simulink model "Fly_By_Wire_Logical_Architecture"  (R2025a)
settings: Solver=VariableStepAuto  StartTime=0.0  StopTime=10.0  RelTol=1e-3
(part 1 of 2)
settings Model: Creator=annic  LastModifiedBy=annic

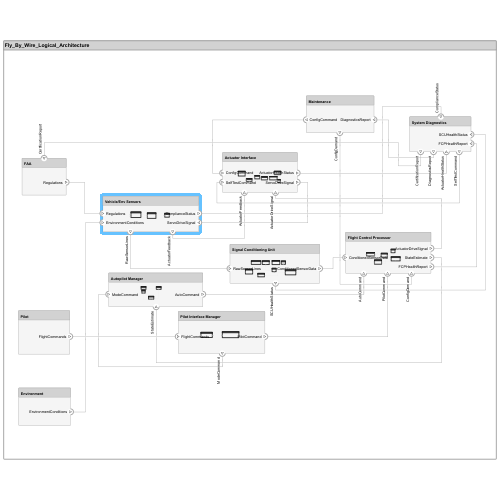
[thumbnail: Simulink's stored preview of the top-level diagram]
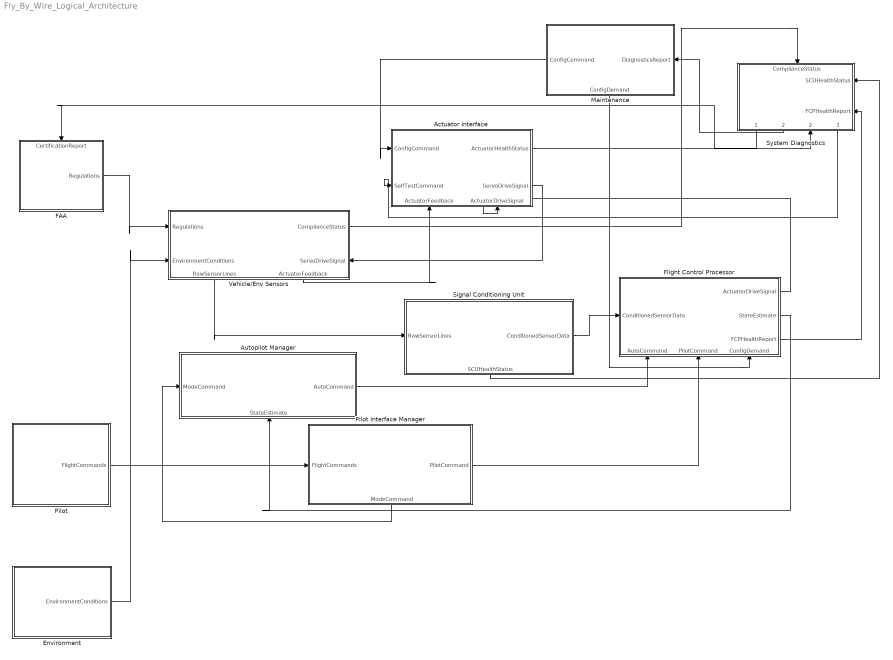
== system Fly_By_Wire_Logical_Architecture ==
  Actuator Interface : Subsystem
      settings: PortSchema="{\"entries\":[{\"content\":{\"headerSize\":26,\"margin\":15,\"minimumSpacing\":25,\"sides\":[{\"content\":{\"connectorIds\":[\"In3\",\"In1\"]},\"type\":\"ConnectorPlacement.EquallySpacedRectSide\",\"uuid\":\"65641699-9f7d-4c29-a70e-9e8ac59d97d8\"},{\"content\":{\"connectorIds\":[\"Out1\",\"Out2\"],\"side\":\"RIGHT\"},\"type\":\"ConnectorPlacement.EquallySpacedRectSide\",\"uuid\":\"1bd5edf9-dcd5-4263-91ef-6bf36c773327\"},{\"content\":{\"side\":\"TOP\"},\"type\":\"ConnectorPlacement.EquallySpacedRectSide\",\"uuid\":\"e3031d72-1a7c-40a3-b76e-c1b9cc4f41a2\"},{\"content\":{\"connectorIds\":[\"In2\",\"In4\"],\"side\":\"BOTTOM\"},\"type\":\"ConnectorPlacement.EquallySpacedRectSide\",\"uuid\":\"36dfb4ef-dbe8-4037-a31c-a1fb1d1c9c8b\"}]},\"type\":\"ConnectorPlacement.EquallySpacedConnector\",\"uuid\":\"735ff59d-d504-4a4c-a5dd-88c988b53692\"}],\"packageUris\":[\"http://schema.mathworks.com/mf0/Connector/R2020b\"],\"version\":\"1.0\"}"
  Autopilot Manager : Subsystem
      settings: PortSchema="{\"entries\":[{\"content\":{\"headerSize\":26,\"margin\":15,\"minimumSpacing\":25,\"sides\":[{\"content\":{\"connectorIds\":[\"In2\"]},\"type\":\"ConnectorPlacement.EquallySpacedRectSide\",\"uuid\":\"65641699-9f7d-4c29-a70e-9e8ac59d97d8\"},{\"content\":{\"connectorIds\":[\"Out1\"],\"side\":\"RIGHT\"},\"type\":\"ConnectorPlacement.EquallySpacedRectSide\",\"uuid\":\"1bd5edf9-dcd5-4263-91ef-6bf36c773327\"},{\"content\":{\"side\":\"TOP\"},\"type\":\"ConnectorPlacement.EquallySpacedRectSide\",\"uuid\":\"e3031d72-1a7c-40a3-b76e-c1b9cc4f41a2\"},{\"content\":{\"connectorIds\":[\"In1\"],\"side\":\"BOTTOM\"},\"type\":\"ConnectorPlacement.EquallySpacedRectSide\",\"uuid\":\"52da988e-5309-44fa-8186-16f50d2bf4d2\"}]},\"type\":\"ConnectorPlacement.EquallySpacedConnector\",\"uuid\":\"735ff59d-d504-4a4c-a5dd-88c988b53692\"}],\"packageUris\":[\"http://schema.mathworks.com/mf0/Connector/R2020b\"],\"version\":\"1.0\"}"
  Environment : Subsystem
      settings: PortSchema="{\"entries\":[{\"content\":{\"headerSize\":26,\"margin\":15,\"minimumSpacing\":25,\"sides\":[{\"content\":{},\"type\":\"ConnectorPlacement.EquallySpacedRectSide\",\"uuid\":\"65641699-9f7d-4c29-a70e-9e8ac59d97d8\"},{\"content\":{\"connectorIds\":[\"Out1\"],\"side\":\"RIGHT\"},\"type\":\"ConnectorPlacement.EquallySpacedRectSide\",\"uuid\":\"1bd5edf9-dcd5-4263-91ef-6bf36c773327\"},{\"content\":{\"side\":\"TOP\"},\"type\":\"ConnectorPlacement.EquallySpacedRectSide\",\"uuid\":\"e3031d72-1a7c-40a3-b76e-c1b9cc4f41a2\"}]},\"type\":\"ConnectorPlacement.EquallySpacedConnector\",\"uuid\":\"735ff59d-d504-4a4c-a5dd-88c988b53692\"}],\"packageUris\":[\"http://schema.mathworks.com/mf0/Connector/R2020b\"],\"version\":\"1.0\"}"
  FAA : Subsystem
      settings: PortSchema="{\"entries\":[{\"content\":{\"headerSize\":26,\"margin\":15,\"minimumSpacing\":25,\"sides\":[{\"content\":{},\"type\":\"ConnectorPlacement.EquallySpacedRectSide\",\"uuid\":\"65641699-9f7d-4c29-a70e-9e8ac59d97d8\"},{\"content\":{\"connectorIds\":[\"Out1\"],\"side\":\"RIGHT\"},\"type\":\"ConnectorPlacement.EquallySpacedRectSide\",\"uuid\":\"1bd5edf9-dcd5-4263-91ef-6bf36c773327\"},{\"content\":{\"connectorIds\":[\"In1\"],\"side\":\"TOP\"},\"type\":\"ConnectorPlacement.EquallySpacedRectSide\",\"uuid\":\"e3031d72-1a7c-40a3-b76e-c1b9cc4f41a2\"}]},\"type\":\"ConnectorPlacement.EquallySpacedConnector\",\"uuid\":\"735ff59d-d504-4a4c-a5dd-88c988b53692\"}],\"packageUris\":[\"http://schema.mathworks.com/mf0/Connector/R2020b\"],\"version\":\"1.0\"}"
  Flight Control Processor : Subsystem
      settings: PortSchema="{\"entries\":[{\"content\":{\"headerSize\":26,\"margin\":15,\"minimumSpacing\":25,\"sides\":[{\"content\":{\"connectorIds\":[\"In4\"]},\"type\":\"ConnectorPlacement.EquallySpacedRectSide\",\"uuid\":\"65641699-9f7d-4c29-a70e-9e8ac59d97d8\"},{\"content\":{\"connectorIds\":[\"Out1\",\"Out2\",\"Out3\"],\"side\":\"RIGHT\"},\"type\":\"ConnectorPlacement.EquallySpacedRectSide\",\"uuid\":\"1bd5edf9-dcd5-4263-91ef-6bf36c773327\"},{\"content\":{\"side\":\"TOP\"},\"type\":\"ConnectorPlacement.EquallySpacedRectSide\",\"uuid\":\"e3031d72-1a7c-40a3-b76e-c1b9cc4f41a2\"},{\"content\":{\"connectorIds\":[\"In1\",\"In2\",\"In3\"],\"side\":\"BOTTOM\"},\"type\":\"ConnectorPlacement.EquallySpacedRectSide\",\"uuid\":\"7b518512-c8fb-468a-b6d8-b7f108893699\"}]},\"type\":\"ConnectorPlacement.EquallySpacedConnector\",\"uuid\":\"735ff59d-d504-4a4c-a5dd-88c988b53692\"}],\"packageUris\":[\"http://schema.mathworks.com/mf0/Connector/R2020b\"],\"version\":\"1.0\"}"
  Maintenance : Subsystem
      settings: PortSchema="{\"entries\":[{\"content\":{\"headerSize\":26,\"margin\":15,\"minimumSpacing\":25,\"sides\":[{\"content\":{\"connectorIds\":[\"Out2\"]},\"type\":\"ConnectorPlacement.EquallySpacedRectSide\",\"uuid\":\"65641699-9f7d-4c29-a70e-9e8ac59d97d8\"},{\"content\":{\"connectorIds\":[\"In1\"],\"side\":\"RIGHT\"},\"type\":\"ConnectorPlacement.EquallySpacedRectSide\",\"uuid\":\"1bd5edf9-dcd5-4263-91ef-6bf36c773327\"},{\"content\":{\"side\":\"TOP\"},\"type\":\"ConnectorPlacement.EquallySpacedRectSide\",\"uuid\":\"e3031d72-1a7c-40a3-b76e-c1b9cc4f41a2\"},{\"content\":{\"connectorIds\":[\"Out1\"],\"side\":\"BOTTOM\"},\"type\":\"ConnectorPlacement.EquallySpacedRectSide\",\"uuid\":\"ea023d6c-f3dd-49c8-b271-fb5b1eb556b6\"}]},\"type\":\"ConnectorPlacement.EquallySpacedConnector\",\"uuid\":\"735ff59d-d504-4a4c-a5dd-88c988b53692\"}],\"packageUris\":[\"http://schema.mathworks.com/mf0/Connector/R2020b\"],\"version\":\"1.0\"}"
  Pilot : Subsystem
      settings: PortSchema="{\"entries\":[{\"content\":{\"headerSize\":26,\"margin\":15,\"minimumSpacing\":25,\"sides\":[{\"content\":{},\"type\":\"ConnectorPlacement.EquallySpacedRectSide\",\"uuid\":\"65641699-9f7d-4c29-a70e-9e8ac59d97d8\"},{\"content\":{\"connectorIds\":[\"Out1\"],\"side\":\"RIGHT\"},\"type\":\"ConnectorPlacement.EquallySpacedRectSide\",\"uuid\":\"1bd5edf9-dcd5-4263-91ef-6bf36c773327\"},{\"content\":{\"side\":\"TOP\"},\"type\":\"ConnectorPlacement.EquallySpacedRectSide\",\"uuid\":\"e3031d72-1a7c-40a3-b76e-c1b9cc4f41a2\"}]},\"type\":\"ConnectorPlacement.EquallySpacedConnector\",\"uuid\":\"735ff59d-d504-4a4c-a5dd-88c988b53692\"}],\"packageUris\":[\"http://schema.mathworks.com/mf0/Connector/R2020b\"],\"version\":\"1.0\"}"
  Pilot Interface Manager : Subsystem
      settings: PortSchema="{\"entries\":[{\"content\":{\"headerSize\":26,\"margin\":15,\"minimumSpacing\":25,\"sides\":[{\"content\":{\"connectorIds\":[\"In1\"]},\"type\":\"ConnectorPlacement.EquallySpacedRectSide\",\"uuid\":\"65641699-9f7d-4c29-a70e-9e8ac59d97d8\"},{\"content\":{\"connectorIds\":[\"Out2\"],\"side\":\"RIGHT\"},\"type\":\"ConnectorPlacement.EquallySpacedRectSide\",\"uuid\":\"1bd5edf9-dcd5-4263-91ef-6bf36c773327\"},{\"content\":{\"side\":\"TOP\"},\"type\":\"ConnectorPlacement.EquallySpacedRectSide\",\"uuid\":\"e3031d72-1a7c-40a3-b76e-c1b9cc4f41a2\"},{\"content\":{\"connectorIds\":[\"Out1\"],\"side\":\"BOTTOM\"},\"type\":\"ConnectorPlacement.EquallySpacedRectSide\",\"uuid\":\"6cbbdc26-ed79-4d1f-9a0d-eece13b623f5\"}]},\"type\":\"ConnectorPlacement.EquallySpacedConnector\",\"uuid\":\"735ff59d-d504-4a4c-a5dd-88c988b53692\"}],\"packageUris\":[\"http://schema.mathworks.com/mf0/Connector/R2020b\"],\"version\":\"1.0\"}"
  Signal Conditioning Unit : Subsystem
      settings: PortSchema="{\"entries\":[{\"content\":{\"headerSize\":26,\"margin\":15,\"minimumSpacing\":25,\"sides\":[{\"content\":{\"connectorIds\":[\"In1\"]},\"type\":\"ConnectorPlacement.EquallySpacedRectSide\",\"uuid\":\"65641699-9f7d-4c29-a70e-9e8ac59d97d8\"},{\"content\":{\"connectorIds\":[\"Out2\"],\"side\":\"RIGHT\"},\"type\":\"ConnectorPlacement.EquallySpacedRectSide\",\"uuid\":\"1bd5edf9-dcd5-4263-91ef-6bf36c773327\"},{\"content\":{\"side\":\"TOP\"},\"type\":\"ConnectorPlacement.EquallySpacedRectSide\",\"uuid\":\"e3031d72-1a7c-40a3-b76e-c1b9cc4f41a2\"},{\"content\":{\"connectorIds\":[\"Out1\"],\"side\":\"BOTTOM\"},\"type\":\"ConnectorPlacement.EquallySpacedRectSide\",\"uuid\":\"ec32d637-ee55-45dc-82dd-59b996a90ff2\"}]},\"type\":\"ConnectorPlacement.EquallySpacedConnector\",\"uuid\":\"735ff59d-d504-4a4c-a5dd-88c988b53692\"}],\"packageUris\":[\"http://schema.mathworks.com/mf0/Connector/R2020b\"],\"version\":\"1.0\"}"
  System Diagnostics : Subsystem
      settings: PortSchema="{\"entries\":[{\"content\":{\"headerSize\":26,\"margin\":15,\"minimumSpacing\":25,\"sides\":[{\"content\":{},\"type\":\"ConnectorPlacement.EquallySpacedRectSide\",\"uuid\":\"65641699-9f7d-4c29-a70e-9e8ac59d97d8\"},{\"content\":{\"connectorIds\":[\"In3\",\"In4\"],\"side\":\"RIGHT\"},\"type\":\"ConnectorPlacement.EquallySpacedRectSide\",\"uuid\":\"1bd5edf9-dcd5-4263-91ef-6bf36c773327\"},{\"content\":{\"connectorIds\":[\"In1\"],\"side\":\"TOP\"},\"type\":\"ConnectorPlacement.EquallySpacedRectSide\",\"uuid\":\"e3031d72-1a7c-40a3-b76e-c1b9cc4f41a2\"},{\"content\":{\"connectorIds\":[\"Out1\",\"Out2\",\"In2\",\"Out3\"],\"side\":\"BOTTOM\"},\"type\":\"ConnectorPlacement.EquallySpacedRectSide\",\"uuid\":\"960bf6e0-3098-4419-abea-36272d90c204\"}]},\"type\":\"ConnectorPlacement.EquallySpacedConnector\",\"uuid\":\"735ff59d-d504-4a4c-a5dd-88c988b53692\"}],\"packageUris\":[\"http://schema.mathworks.com/mf0/Connector/R2020b\"],\"version\":\"1.0\"}"
  Vehicle/Env Sensors : Subsystem
      settings: PortSchema="{\"entries\":[{\"content\":{\"headerSize\":26,\"margin\":15,\"minimumSpacing\":25,\"sides\":[{\"content\":{\"connectorIds\":[\"In1\",\"In2\"]},\"type\":\"ConnectorPlacement.EquallySpacedRectSide\",\"uuid\":\"65641699-9f7d-4c29-a70e-9e8ac59d97d8\"},{\"content\":{\"connectorIds\":[\"Out1\",\"In3\"],\"side\":\"RIGHT\"},\"type\":\"ConnectorPlacement.EquallySpacedRectSide\",\"uuid\":\"1bd5edf9-dcd5-4263-91ef-6bf36c773327\"},{\"content\":{\"side\":\"TOP\"},\"type\":\"ConnectorPlacement.EquallySpacedRectSide\",\"uuid\":\"e3031d72-1a7c-40a3-b76e-c1b9cc4f41a2\"},{\"content\":{\"connectorIds\":[\"Out2\",\"Out3\"],\"side\":\"BOTTOM\"},\"type\":\"ConnectorPlacement.EquallySpacedRectSide\",\"uuid\":\"8c0a4771-f010-4a1b-a319-a816648614b3\"}]},\"type\":\"ConnectorPlacement.EquallySpacedConnector\",\"uuid\":\"735ff59d-d504-4a4c-a5dd-88c988b53692\"}],\"packageUris\":[\"http://schema.mathworks.com/mf0/Connector/R2020b\"],\"version\":\"1.0\"}"
  wires:
  Pilot/1(FlightCommands) -> Pilot Interface Manager/1(FlightCommands)
  Pilot Interface Manager/2(PilotCommand) -> Flight Control Processor/2(PilotCommand)
  Signal Conditioning Unit/2(ConditionedSensorData) -> Flight Control Processor/4(ConditionedSensorData)
  Flight Control Processor/3(FCPHealthReport) -> System Diagnostics/4(FCPHealthReport)
  Actuator Interface/2(ServoDriveSignal) -> Vehicle/Env Sensors/3(ServoDriveSignal)
  FAA/1(Regulations) -> Vehicle/Env Sensors/1(Regulations)
  Maintenance/1(ConfigDemand) -> Flight Control Processor/3(ConfigDemand)
  Pilot Interface Manager/1(ModeCommand) -> Autopilot Manager/2(ModeCommand)
  Autopilot Manager/1(AutoCommand) -> Flight Control Processor/1(AutoCommand)
  Flight Control Processor/1(ActuatorDriveSignal) -> Actuator Interface/4(ActuatorDriveSignal)
  Vehicle/Env Sensors/2(RawSensorLines) -> Signal Conditioning Unit/1(RawSensorLines)
  Flight Control Processor/2(StateEstimate) -> Autopilot Manager/1(StateEstimate)
  Maintenance/2(ConfigCommand) -> Actuator Interface/3(ConfigCommand)
  Vehicle/Env Sensors/3(ActuatorFeedback) -> Actuator Interface/2(ActuatorFeedback)
  Signal Conditioning Unit/1(SCUHealthStatus) -> System Diagnostics/3(SCUHealthStatus)
  System Diagnostics/3(SelfTestCommand) -> Actuator Interface/1(SelfTestCommand)
  Actuator Interface/1(ActuatorHealthStatus) -> System Diagnostics/2(ActuatorHealthStatus)
  System Diagnostics/2(DiagnosticsReport) -> Maintenance/1(DiagnosticsReport)
  System Diagnostics/1(CertificationReport) -> FAA/1(CertificationReport)
  Environment/1(EnvironmentConditions) -> Vehicle/Env Sensors/2(EnvironmentConditions)
  Vehicle/Env Sensors/1(ComplianceStatus) -> System Diagnostics/1(ComplianceStatus)

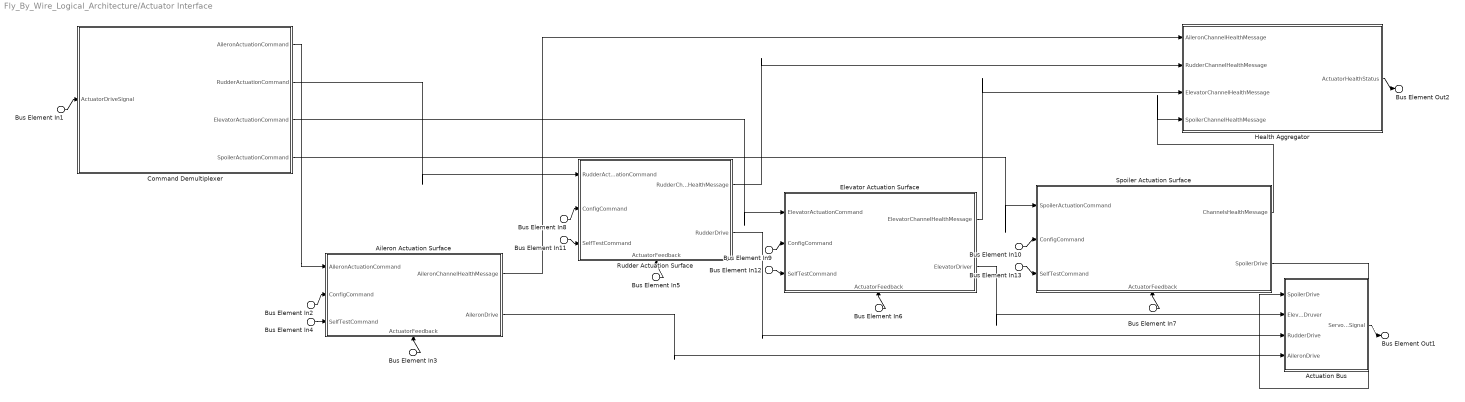
== system Fly_By_Wire_Logical_Architecture/Actuator Interface ==
  Bus Element In{4,11..13} (4 alike) : Inport  PortName=SelfTestCommand
  Bus Element In{3,5..7} (4 alike) : Inport  Port=2  PortName=ActuatorFeedback
  Bus Element In{2,8..10} (4 alike) : Inport  Port=3  PortName=ConfigCommand
  Bus Element In1 : Inport  Port=4  PortName=ActuatorDriveSignal
  Actuation Bus : Subsystem
      settings: PortSchema="{\"entries\":[{\"content\":{\"headerSize\":26,\"margin\":15,\"minimumSpacing\":25,\"sides\":[{\"content\":{\"connectorIds\":[\"In1\",\"In2\",\"In3\",\"In4\"]},\"type\":\"ConnectorPlacement.EquallySpacedRectSide\",\"uuid\":\"ba076da3-00e0-45ec-8905-3337491584c0\"},{\"content\":{\"connectorIds\":[\"Out1\"],\"side\":\"RIGHT\"},\"type\":\"ConnectorPlacement.EquallySpacedRectSide\",\"uuid\":\"72ac928f-e9a5-49d3-a941-8254f9ba21ee\"},{\"content\":{\"side\":\"TOP\"},\"type\":\"ConnectorPlacement.EquallySpacedRectSide\",\"uuid\":\"2a7ce638-5f70-4cef-9a31-c53717642639\"}]},\"type\":\"ConnectorPlacement.EquallySpacedConnector\",\"uuid\":\"ee460f65-3357-4135-aa65-636d7831ce3e\"}],\"packageUris\":[\"http://schema.mathworks.com/mf0/Connector/R2020b\"],\"version\":\"1.0\"}"
  Aileron Actuation Surface : Subsystem
      settings: PortSchema="{\"entries\":[{\"content\":{\"headerSize\":26,\"margin\":15,\"minimumSpacing\":25,\"sides\":[{\"content\":{\"connectorIds\":[\"In1\",\"In2\",\"In3\"]},\"type\":\"ConnectorPlacement.EquallySpacedRectSide\",\"uuid\":\"ba076da3-00e0-45ec-8905-3337491584c0\"},{\"content\":{\"connectorIds\":[\"Out1\",\"Out2\"],\"side\":\"RIGHT\"},\"type\":\"ConnectorPlacement.EquallySpacedRectSide\",\"uuid\":\"72ac928f-e9a5-49d3-a941-8254f9ba21ee\"},{\"content\":{\"side\":\"TOP\"},\"type\":\"ConnectorPlacement.EquallySpacedRectSide\",\"uuid\":\"2a7ce638-5f70-4cef-9a31-c53717642639\"},{\"content\":{\"connectorIds\":[\"In4\"],\"side\":\"BOTTOM\"},\"type\":\"ConnectorPlacement.EquallySpacedRectSide\",\"uuid\":\"37b8f7a7-18c8-44ab-b4f9-2047c5c4ee6a\"}]},\"type\":\"ConnectorPlacement.EquallySpacedConnector\",\"uuid\":\"ee460f65-3357-4135-aa65-636d7831ce3e\"}],\"packageUris\":[\"http://schema.mathworks.com/mf0/Connector/R2020b\"],\"version\":\"1.0\"}"
  Command Demultiplexer : Subsystem
      settings: PortSchema="{\"entries\":[{\"content\":{\"headerSize\":26,\"margin\":15,\"minimumSpacing\":25,\"sides\":[{\"content\":{\"connectorIds\":[\"In1\"]},\"type\":\"ConnectorPlacement.EquallySpacedRectSide\",\"uuid\":\"ba076da3-00e0-45ec-8905-3337491584c0\"},{\"content\":{\"connectorIds\":[\"Out1\",\"Out2\",\"Out3\",\"Out4\"],\"side\":\"RIGHT\"},\"type\":\"ConnectorPlacement.EquallySpacedRectSide\",\"uuid\":\"72ac928f-e9a5-49d3-a941-8254f9ba21ee\"},{\"content\":{\"side\":\"TOP\"},\"type\":\"ConnectorPlacement.EquallySpacedRectSide\",\"uuid\":\"2a7ce638-5f70-4cef-9a31-c53717642639\"}]},\"type\":\"ConnectorPlacement.EquallySpacedConnector\",\"uuid\":\"ee460f65-3357-4135-aa65-636d7831ce3e\"}],\"packageUris\":[\"http://schema.mathworks.com/mf0/Connector/R2020b\"],\"version\":\"1.0\"}"
  Elevator Actuation Surface : Subsystem
      settings: PortSchema="{\"entries\":[{\"content\":{\"headerSize\":26,\"margin\":15,\"minimumSpacing\":25,\"sides\":[{\"content\":{\"connectorIds\":[\"In1\",\"In2\",\"In3\"]},\"type\":\"ConnectorPlacement.EquallySpacedRectSide\",\"uuid\":\"ba076da3-00e0-45ec-8905-3337491584c0\"},{\"content\":{\"connectorIds\":[\"Out1\",\"Out2\"],\"side\":\"RIGHT\"},\"type\":\"ConnectorPlacement.EquallySpacedRectSide\",\"uuid\":\"72ac928f-e9a5-49d3-a941-8254f9ba21ee\"},{\"content\":{\"side\":\"TOP\"},\"type\":\"ConnectorPlacement.EquallySpacedRectSide\",\"uuid\":\"2a7ce638-5f70-4cef-9a31-c53717642639\"},{\"content\":{\"connectorIds\":[\"In4\"],\"side\":\"BOTTOM\"},\"type\":\"ConnectorPlacement.EquallySpacedRectSide\",\"uuid\":\"da968ea3-538c-4f8d-b054-92697d47904c\"}]},\"type\":\"ConnectorPlacement.EquallySpacedConnector\",\"uuid\":\"ee460f65-3357-4135-aa65-636d7831ce3e\"}],\"packageUris\":[\"http://schema.mathworks.com/mf0/Connector/R2020b\"],\"version\":\"1.0\"}"
  Health Aggregator : Subsystem
      settings: PortSchema="{\"entries\":[{\"content\":{\"headerSize\":26,\"margin\":15,\"minimumSpacing\":25,\"sides\":[{\"content\":{\"connectorIds\":[\"In1\",\"In2\",\"In3\",\"In4\"]},\"type\":\"ConnectorPlacement.EquallySpacedRectSide\",\"uuid\":\"ba076da3-00e0-45ec-8905-3337491584c0\"},{\"content\":{\"connectorIds\":[\"Out1\"],\"side\":\"RIGHT\"},\"type\":\"ConnectorPlacement.EquallySpacedRectSide\",\"uuid\":\"72ac928f-e9a5-49d3-a941-8254f9ba21ee\"},{\"content\":{\"side\":\"TOP\"},\"type\":\"ConnectorPlacement.EquallySpacedRectSide\",\"uuid\":\"2a7ce638-5f70-4cef-9a31-c53717642639\"}]},\"type\":\"ConnectorPlacement.EquallySpacedConnector\",\"uuid\":\"ee460f65-3357-4135-aa65-636d7831ce3e\"}],\"packageUris\":[\"http://schema.mathworks.com/mf0/Connector/R2020b\"],\"version\":\"1.0\"}"
  Rudder Actuation Surface : Subsystem
      settings: PortSchema="{\"entries\":[{\"content\":{\"headerSize\":26,\"margin\":15,\"minimumSpacing\":25,\"sides\":[{\"content\":{\"connectorIds\":[\"In1\",\"In2\",\"In3\"]},\"type\":\"ConnectorPlacement.EquallySpacedRectSide\",\"uuid\":\"ba076da3-00e0-45ec-8905-3337491584c0\"},{\"content\":{\"connectorIds\":[\"Out1\",\"Out2\"],\"side\":\"RIGHT\"},\"type\":\"ConnectorPlacement.EquallySpacedRectSide\",\"uuid\":\"72ac928f-e9a5-49d3-a941-8254f9ba21ee\"},{\"content\":{\"side\":\"TOP\"},\"type\":\"ConnectorPlacement.EquallySpacedRectSide\",\"uuid\":\"2a7ce638-5f70-4cef-9a31-c53717642639\"},{\"content\":{\"connectorIds\":[\"In4\"],\"side\":\"BOTTOM\"},\"type\":\"ConnectorPlacement.EquallySpacedRectSide\",\"uuid\":\"cf85ff21-1305-4281-a344-bee9168b9325\"}]},\"type\":\"ConnectorPlacement.EquallySpacedConnector\",\"uuid\":\"ee460f65-3357-4135-aa65-636d7831ce3e\"}],\"packageUris\":[\"http://schema.mathworks.com/mf0/Connector/R2020b\"],\"version\":\"1.0\"}"
  Spoiler Actuation Surface : Subsystem
      settings: PortSchema="{\"entries\":[{\"content\":{\"headerSize\":26,\"margin\":15,\"minimumSpacing\":25,\"sides\":[{\"content\":{\"connectorIds\":[\"In1\",\"In2\",\"In3\"]},\"type\":\"ConnectorPlacement.EquallySpacedRectSide\",\"uuid\":\"ba076da3-00e0-45ec-8905-3337491584c0\"},{\"content\":{\"connectorIds\":[\"Out1\",\"Out2\"],\"side\":\"RIGHT\"},\"type\":\"ConnectorPlacement.EquallySpacedRectSide\",\"uuid\":\"72ac928f-e9a5-49d3-a941-8254f9ba21ee\"},{\"content\":{\"side\":\"TOP\"},\"type\":\"ConnectorPlacement.EquallySpacedRectSide\",\"uuid\":\"2a7ce638-5f70-4cef-9a31-c53717642639\"},{\"content\":{\"connectorIds\":[\"In4\"],\"side\":\"BOTTOM\"},\"type\":\"ConnectorPlacement.EquallySpacedRectSide\",\"uuid\":\"fb37be59-469d-422c-9393-ca605343550b\"}]},\"type\":\"ConnectorPlacement.EquallySpacedConnector\",\"uuid\":\"ee460f65-3357-4135-aa65-636d7831ce3e\"}],\"packageUris\":[\"http://schema.mathworks.com/mf0/Connector/R2020b\"],\"version\":\"1.0\"}"
  Bus Element Out2 : Outport  PortName=ActuatorHealthStatus
  Bus Element Out1 : Outport  Port=2  PortName=ServoDriveSignal
  wires:
  Bus Element In1/1 -> Command Demultiplexer/1(ActuatorDriveSignal)
  Command Demultiplexer/3(ElevatorActuationCommand) -> Elevator Actuation Surface/1(ElevatorActuationCommand)
  Command Demultiplexer/1(AileronActuationCommand) -> Aileron Actuation Surface/1(AileronActuationCommand)
  Command Demultiplexer/2(RudderActuationCommand) -> Rudder Actuation Surface/1(RudderActuationCommand)
  Command Demultiplexer/4(SpoilerActuationCommand) -> Spoiler Actuation Surface/1(SpoilerActuationCommand)
  Health Aggregator/1(ActuatorHealthStatus) -> Bus Element Out2/1
  Bus Element In3/1 -> Aileron Actuation Surface/4(ActuatorFeedback)
  Bus Element In5/1 -> Rudder Actuation Surface/4(ActuatorFeedback)
  Bus Element In6/1 -> Elevator Actuation Surface/4(ActuatorFeedback)
  Bus Element In7/1 -> Spoiler Actuation Surface/4(ActuatorFeedback)
  Spoiler Actuation Surface/2(SpoilerDrive) -> Actuation Bus/1(SpoilerDrive)
  Elevator Actuation Surface/2(ElevatorDriver) -> Actuation Bus/2(ElevatorDruver)
  Rudder Actuation Surface/2(RudderDrive) -> Actuation Bus/3(RudderDrive)
  Aileron Actuation Surface/2(AileronDrive) -> Actuation Bus/4(AileronDrive)
  Actuation Bus/1(ServoDriveSignal) -> Bus Element Out1/1
  Spoiler Actuation Surface/1(ChannelsHealthMessage) -> Health Aggregator/4(SpoilerChannelHealthMessage)
  Elevator Actuation Surface/1(ElevatorChannelHealthMessage) -> Health Aggregator/3(ElevatorChannelHealthMessage)
  Rudder Actuation Surface/1(RudderChannelHealthMessage) -> Health Aggregator/2(RudderChannelHealthMessage)
  Aileron Actuation Surface/1(AileronChannelHealthMessage) -> Health Aggregator/1(AileronChannelHealthMessage)
  Bus Element In2/1 -> Aileron Actuation Surface/2(ConfigCommand)
  Bus Element In8/1 -> Rudder Actuation Surface/2(ConfigCommand)
  Bus Element In9/1 -> Elevator Actuation Surface/2(ConfigCommand)
  Bus Element In10/1 -> Spoiler Actuation Surface/2(ConfigCommand)
  Bus Element In4/1 -> Aileron Actuation Surface/3(SelfTestCommand)
  Bus Element In11/1 -> Rudder Actuation Surface/3(SelfTestCommand)
  Bus Element In12/1 -> Elevator Actuation Surface/3(SelfTestCommand)
  Bus Element In13/1 -> Spoiler Actuation Surface/3(SelfTestCommand)

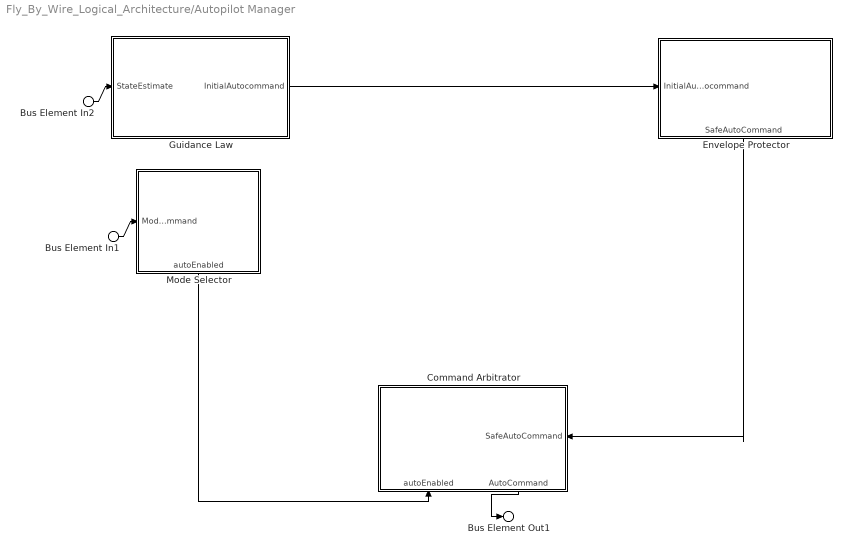
== system Fly_By_Wire_Logical_Architecture/Autopilot Manager ==
  Bus Element In2 : Inport  PortName=StateEstimate
  Bus Element In1 : Inport  Port=2  PortName=ModeCommand
  Command Arbitrator : Subsystem
      settings: PortSchema="{\"entries\":[{\"content\":{\"headerSize\":26,\"margin\":15,\"minimumSpacing\":25,\"sides\":[{\"content\":{},\"type\":\"ConnectorPlacement.EquallySpacedRectSide\",\"uuid\":\"ba076da3-00e0-45ec-8905-3337491584c0\"},{\"content\":{\"connectorIds\":[\"In1\"],\"side\":\"RIGHT\"},\"type\":\"ConnectorPlacement.EquallySpacedRectSide\",\"uuid\":\"72ac928f-e9a5-49d3-a941-8254f9ba21ee\"},{\"content\":{\"side\":\"TOP\"},\"type\":\"ConnectorPlacement.EquallySpacedRectSide\",\"uuid\":\"2a7ce638-5f70-4cef-9a31-c53717642639\"},{\"content\":{\"connectorIds\":[\"In2\",\"Out1\"],\"side\":\"BOTTOM\"},\"type\":\"ConnectorPlacement.EquallySpacedRectSide\",\"uuid\":\"1a7ca1cc-0da0-4af6-a72e-3b6283aa0633\"}]},\"type\":\"ConnectorPlacement.EquallySpacedConnector\",\"uuid\":\"ee460f65-3357-4135-aa65-636d7831ce3e\"}],\"packageUris\":[\"http://schema.mathworks.com/mf0/Connector/R2020b\"],\"version\":\"1.0\"}"
  Envelope Protector : Subsystem
      settings: PortSchema="{\"entries\":[{\"content\":{\"headerSize\":26,\"margin\":15,\"minimumSpacing\":25,\"sides\":[{\"content\":{\"connectorIds\":[\"In1\"]},\"type\":\"ConnectorPlacement.EquallySpacedRectSide\",\"uuid\":\"ba076da3-00e0-45ec-8905-3337491584c0\"},{\"content\":{\"side\":\"RIGHT\"},\"type\":\"ConnectorPlacement.EquallySpacedRectSide\",\"uuid\":\"72ac928f-e9a5-49d3-a941-8254f9ba21ee\"},{\"content\":{\"side\":\"TOP\"},\"type\":\"ConnectorPlacement.EquallySpacedRectSide\",\"uuid\":\"2a7ce638-5f70-4cef-9a31-c53717642639\"},{\"content\":{\"connectorIds\":[\"Out1\"],\"side\":\"BOTTOM\"},\"type\":\"ConnectorPlacement.EquallySpacedRectSide\",\"uuid\":\"aec99c5b-079c-44bf-99cb-705dd22d0283\"}]},\"type\":\"ConnectorPlacement.EquallySpacedConnector\",\"uuid\":\"ee460f65-3357-4135-aa65-636d7831ce3e\"}],\"packageUris\":[\"http://schema.mathworks.com/mf0/Connector/R2020b\"],\"version\":\"1.0\"}"
  Guidance Law : Subsystem
      settings: PortSchema="{\"entries\":[{\"content\":{\"headerSize\":26,\"margin\":15,\"minimumSpacing\":25,\"sides\":[{\"content\":{\"connectorIds\":[\"In1\"]},\"type\":\"ConnectorPlacement.EquallySpacedRectSide\",\"uuid\":\"ba076da3-00e0-45ec-8905-3337491584c0\"},{\"content\":{\"connectorIds\":[\"Out1\"],\"side\":\"RIGHT\"},\"type\":\"ConnectorPlacement.EquallySpacedRectSide\",\"uuid\":\"72ac928f-e9a5-49d3-a941-8254f9ba21ee\"},{\"content\":{\"side\":\"TOP\"},\"type\":\"ConnectorPlacement.EquallySpacedRectSide\",\"uuid\":\"2a7ce638-5f70-4cef-9a31-c53717642639\"}]},\"type\":\"ConnectorPlacement.EquallySpacedConnector\",\"uuid\":\"ee460f65-3357-4135-aa65-636d7831ce3e\"}],\"packageUris\":[\"http://schema.mathworks.com/mf0/Connector/R2020b\"],\"version\":\"1.0\"}"
  Mode Selector : Subsystem
      settings: PortSchema="{\"entries\":[{\"content\":{\"headerSize\":26,\"margin\":15,\"minimumSpacing\":25,\"sides\":[{\"content\":{\"connectorIds\":[\"In1\"]},\"type\":\"ConnectorPlacement.EquallySpacedRectSide\",\"uuid\":\"ba076da3-00e0-45ec-8905-3337491584c0\"},{\"content\":{\"side\":\"RIGHT\"},\"type\":\"ConnectorPlacement.EquallySpacedRectSide\",\"uuid\":\"72ac928f-e9a5-49d3-a941-8254f9ba21ee\"},{\"content\":{\"side\":\"TOP\"},\"type\":\"ConnectorPlacement.EquallySpacedRectSide\",\"uuid\":\"2a7ce638-5f70-4cef-9a31-c53717642639\"},{\"content\":{\"connectorIds\":[\"Out1\"],\"side\":\"BOTTOM\"},\"type\":\"ConnectorPlacement.EquallySpacedRectSide\",\"uuid\":\"8e73495f-d2a4-48c3-8f62-4e434c9fd552\"}]},\"type\":\"ConnectorPlacement.EquallySpacedConnector\",\"uuid\":\"ee460f65-3357-4135-aa65-636d7831ce3e\"}],\"packageUris\":[\"http://schema.mathworks.com/mf0/Connector/R2020b\"],\"version\":\"1.0\"}"
  Bus Element Out1 : Outport  PortName=AutoCommand
  wires:
  Bus Element In1/1 -> Mode Selector/1(ModeCommand)
  Mode Selector/1(autoEnabled) -> Command Arbitrator/2(autoEnabled)
  Bus Element In2/1 -> Guidance Law/1(StateEstimate)
  Guidance Law/1(InitialAutocommand) -> Envelope Protector/1(InitialAutocommand)
  Envelope Protector/1(SafeAutoCommand) -> Command Arbitrator/1(SafeAutoCommand)
  Command Arbitrator/1(AutoCommand) -> Bus Element Out1/1

== system Fly_By_Wire_Logical_Architecture/Environment ==
  Bus Element Out1 : Outport  PortName=EnvironmentConditions

== system Fly_By_Wire_Logical_Architecture/FAA ==
  Bus Element In1 : Inport  PortName=CertificationReport
  Bus Element Out1 : Outport  PortName=Regulations

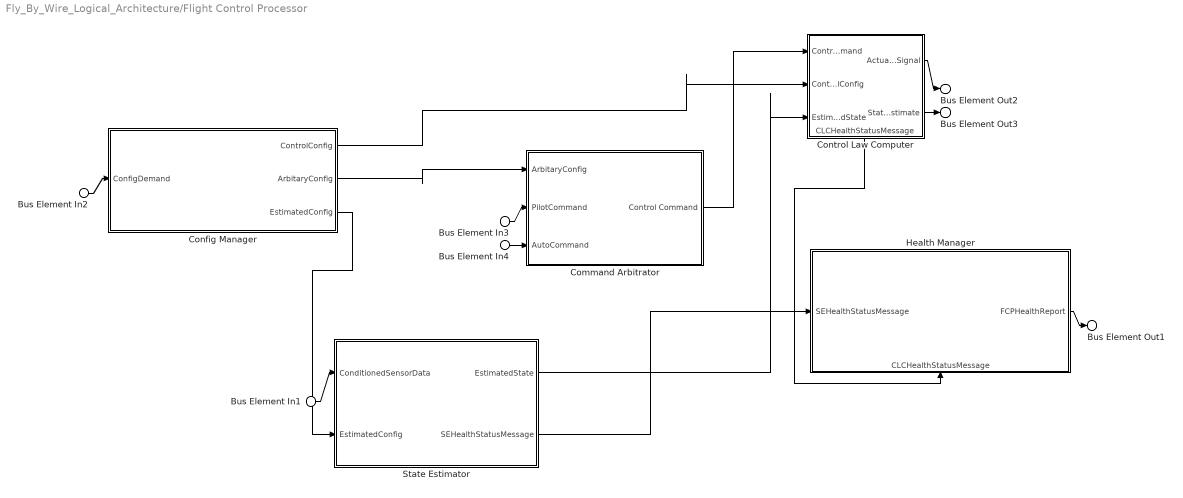
== system Fly_By_Wire_Logical_Architecture/Flight Control Processor ==
  Bus Element In4 : Inport  PortName=AutoCommand
  Bus Element In3 : Inport  Port=2  PortName=PilotCommand
  Bus Element In2 : Inport  Port=3  PortName=ConfigDemand
  Bus Element In1 : Inport  Port=4  PortName=ConditionedSensorData
  Command Arbitrator : Subsystem
      settings: PortSchema="{\"entries\":[{\"content\":{\"headerSize\":26,\"margin\":15,\"minimumSpacing\":25,\"sides\":[{\"content\":{\"connectorIds\":[\"In1\",\"In2\",\"In3\"]},\"type\":\"ConnectorPlacement.EquallySpacedRectSide\",\"uuid\":\"ba076da3-00e0-45ec-8905-3337491584c0\"},{\"content\":{\"connectorIds\":[\"Out1\"],\"side\":\"RIGHT\"},\"type\":\"ConnectorPlacement.EquallySpacedRectSide\",\"uuid\":\"72ac928f-e9a5-49d3-a941-8254f9ba21ee\"},{\"content\":{\"side\":\"TOP\"},\"type\":\"ConnectorPlacement.EquallySpacedRectSide\",\"uuid\":\"2a7ce638-5f70-4cef-9a31-c53717642639\"}]},\"type\":\"ConnectorPlacement.EquallySpacedConnector\",\"uuid\":\"ee460f65-3357-4135-aa65-636d7831ce3e\"}],\"packageUris\":[\"http://schema.mathworks.com/mf0/Connector/R2020b\"],\"version\":\"1.0\"}"
  Config Manager : Subsystem
      settings: PortSchema="{\"entries\":[{\"content\":{\"headerSize\":26,\"margin\":15,\"minimumSpacing\":25,\"sides\":[{\"content\":{\"connectorIds\":[\"In1\"]},\"type\":\"ConnectorPlacement.EquallySpacedRectSide\",\"uuid\":\"ba076da3-00e0-45ec-8905-3337491584c0\"},{\"content\":{\"connectorIds\":[\"Out1\",\"Out2\",\"Out3\"],\"side\":\"RIGHT\"},\"type\":\"ConnectorPlacement.EquallySpacedRectSide\",\"uuid\":\"72ac928f-e9a5-49d3-a941-8254f9ba21ee\"},{\"content\":{\"side\":\"TOP\"},\"type\":\"ConnectorPlacement.EquallySpacedRectSide\",\"uuid\":\"2a7ce638-5f70-4cef-9a31-c53717642639\"}]},\"type\":\"ConnectorPlacement.EquallySpacedConnector\",\"uuid\":\"ee460f65-3357-4135-aa65-636d7831ce3e\"}],\"packageUris\":[\"http://schema.mathworks.com/mf0/Connector/R2020b\"],\"version\":\"1.0\"}"
  Control Law Computer : Subsystem
      settings: PortSchema="{\"entries\":[{\"content\":{\"headerSize\":26,\"margin\":15,\"minimumSpacing\":25,\"sides\":[{\"content\":{\"connectorIds\":[\"In1\",\"In2\",\"In3\"]},\"type\":\"ConnectorPlacement.EquallySpacedRectSide\",\"uuid\":\"ba076da3-00e0-45ec-8905-3337491584c0\"},{\"content\":{\"connectorIds\":[\"Out2\",\"Out3\"],\"side\":\"RIGHT\"},\"type\":\"ConnectorPlacement.EquallySpacedRectSide\",\"uuid\":\"72ac928f-e9a5-49d3-a941-8254f9ba21ee\"},{\"content\":{\"side\":\"TOP\"},\"type\":\"ConnectorPlacement.EquallySpacedRectSide\",\"uuid\":\"2a7ce638-5f70-4cef-9a31-c53717642639\"},{\"content\":{\"connectorIds\":[\"Out1\"],\"side\":\"BOTTOM\"},\"type\":\"ConnectorPlacement.EquallySpacedRectSide\",\"uuid\":\"bd4e1cb1-f676-48c6-817c-282ad026f374\"}]},\"type\":\"ConnectorPlacement.EquallySpacedConnector\",\"uuid\":\"ee460f65-3357-4135-aa65-636d7831ce3e\"}],\"packageUris\":[\"http://schema.mathworks.com/mf0/Connector/R2020b\"],\"version\":\"1.0\"}"
  Health Manager : Subsystem
      settings: PortSchema="{\"entries\":[{\"content\":{\"headerSize\":26,\"margin\":15,\"minimumSpacing\":25,\"sides\":[{\"content\":{\"connectorIds\":[\"In2\"]},\"type\":\"ConnectorPlacement.EquallySpacedRectSide\",\"uuid\":\"ba076da3-00e0-45ec-8905-3337491584c0\"},{\"content\":{\"connectorIds\":[\"Out1\"],\"side\":\"RIGHT\"},\"type\":\"ConnectorPlacement.EquallySpacedRectSide\",\"uuid\":\"72ac928f-e9a5-49d3-a941-8254f9ba21ee\"},{\"content\":{\"side\":\"TOP\"},\"type\":\"ConnectorPlacement.EquallySpacedRectSide\",\"uuid\":\"2a7ce638-5f70-4cef-9a31-c53717642639\"},{\"content\":{\"connectorIds\":[\"In1\"],\"side\":\"BOTTOM\"},\"type\":\"ConnectorPlacement.EquallySpacedRectSide\",\"uuid\":\"e24b6971-791c-4915-a611-182ed08b3073\"}]},\"type\":\"ConnectorPlacement.EquallySpacedConnector\",\"uuid\":\"ee460f65-3357-4135-aa65-636d7831ce3e\"}],\"packageUris\":[\"http://schema.mathworks.com/mf0/Connector/R2020b\"],\"version\":\"1.0\"}"
  State Estimator : Subsystem
      settings: PortSchema="{\"entries\":[{\"content\":{\"headerSize\":26,\"margin\":15,\"minimumSpacing\":25,\"sides\":[{\"content\":{\"connectorIds\":[\"In1\",\"In2\"]},\"type\":\"ConnectorPlacement.EquallySpacedRectSide\",\"uuid\":\"ba076da3-00e0-45ec-8905-3337491584c0\"},{\"content\":{\"connectorIds\":[\"Out1\",\"Out2\"],\"side\":\"RIGHT\"},\"type\":\"ConnectorPlacement.EquallySpacedRectSide\",\"uuid\":\"72ac928f-e9a5-49d3-a941-8254f9ba21ee\"},{\"content\":{\"side\":\"TOP\"},\"type\":\"ConnectorPlacement.EquallySpacedRectSide\",\"uuid\":\"2a7ce638-5f70-4cef-9a31-c53717642639\"}]},\"type\":\"ConnectorPlacement.EquallySpacedConnector\",\"uuid\":\"ee460f65-3357-4135-aa65-636d7831ce3e\"}],\"packageUris\":[\"http://schema.mathworks.com/mf0/Connector/R2020b\"],\"version\":\"1.0\"}"
  Bus Element Out2 : Outport  PortName=ActuatorDriveSignal
  Bus Element Out3 : Outport  Port=2  PortName=StateEstimate
  Bus Element Out1 : Outport  Port=3  PortName=FCPHealthReport
  wires:
  Bus Element In2/1 -> Config Manager/1(ConfigDemand)
  Config Manager/2(ArbitaryConfig) -> Command Arbitrator/1(ArbitaryConfig)
  Config Manager/3(EstimatedConfig) -> State Estimator/2(EstimatedConfig)
  Config Manager/1(ControlConfig) -> Control Law Computer/2(ControlConfig)
  Bus Element In3/1 -> Command Arbitrator/2(PilotCommand)
  Bus Element In4/1 -> Command Arbitrator/3(AutoCommand)
  Command Arbitrator/1(Control Command) -> Control Law Computer/1(ControlCommand)
  Bus Element In1/1 -> State Estimator/1(ConditionedSensorData)
  State Estimator/2(SEHealthStatusMessage) -> Health Manager/2(SEHealthStatusMessage)
  State Estimator/1(EstimatedState) -> Control Law Computer/3(EstimatedState)
  Control Law Computer/2(ActuatorDriveSignal) -> Bus Element Out2/1
  Control Law Computer/3(StateEstimate) -> Bus Element Out3/1
  Health Manager/1(FCPHealthReport) -> Bus Element Out1/1
  Control Law Computer/1(CLCHealthStatusMessage) -> Health Manager/1(CLCHealthStatusMessage)

== system Fly_By_Wire_Logical_Architecture/Maintenance ==
  Bus Element In1 : Inport  PortName=DiagnosticsReport
  Bus Element Out3 : Outport  PortName=ConfigDemand
  Bus Element Out2 : Outport  Port=2  PortName=ConfigCommand

== system Fly_By_Wire_Logical_Architecture/Pilot ==
  Bus Element Out1 : Outport  PortName=FlightCommands

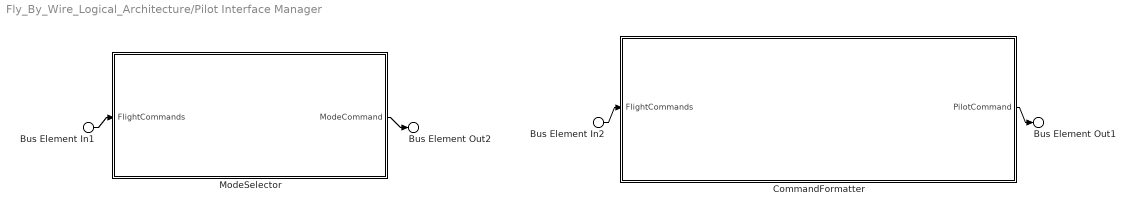
== system Fly_By_Wire_Logical_Architecture/Pilot Interface Manager ==
  Bus Element In1 : Inport  PortName=FlightCommands
  Bus Element In2 : Inport  PortName=FlightCommands
  CommandFormatter : Subsystem
      settings: PortSchema="{\"entries\":[{\"content\":{\"headerSize\":26,\"margin\":15,\"minimumSpacing\":25,\"sides\":[{\"content\":{\"connectorIds\":[\"In1\"]},\"type\":\"ConnectorPlacement.EquallySpacedRectSide\",\"uuid\":\"ba076da3-00e0-45ec-8905-3337491584c0\"},{\"content\":{\"connectorIds\":[\"Out1\"],\"side\":\"RIGHT\"},\"type\":\"ConnectorPlacement.EquallySpacedRectSide\",\"uuid\":\"72ac928f-e9a5-49d3-a941-8254f9ba21ee\"},{\"content\":{\"side\":\"TOP\"},\"type\":\"ConnectorPlacement.EquallySpacedRectSide\",\"uuid\":\"2a7ce638-5f70-4cef-9a31-c53717642639\"}]},\"type\":\"ConnectorPlacement.EquallySpacedConnector\",\"uuid\":\"ee460f65-3357-4135-aa65-636d7831ce3e\"}],\"packageUris\":[\"http://schema.mathworks.com/mf0/Connector/R2020b\"],\"version\":\"1.0\"}"
  ModeSelector : Subsystem
      settings: PortSchema="{\"entries\":[{\"content\":{\"headerSize\":26,\"margin\":15,\"minimumSpacing\":25,\"sides\":[{\"content\":{\"connectorIds\":[\"In1\"]},\"type\":\"ConnectorPlacement.EquallySpacedRectSide\",\"uuid\":\"ba076da3-00e0-45ec-8905-3337491584c0\"},{\"content\":{\"connectorIds\":[\"Out1\"],\"side\":\"RIGHT\"},\"type\":\"ConnectorPlacement.EquallySpacedRectSide\",\"uuid\":\"72ac928f-e9a5-49d3-a941-8254f9ba21ee\"},{\"content\":{\"side\":\"TOP\"},\"type\":\"ConnectorPlacement.EquallySpacedRectSide\",\"uuid\":\"2a7ce638-5f70-4cef-9a31-c53717642639\"}]},\"type\":\"ConnectorPlacement.EquallySpacedConnector\",\"uuid\":\"ee460f65-3357-4135-aa65-636d7831ce3e\"}],\"packageUris\":[\"http://schema.mathworks.com/mf0/Connector/R2020b\"],\"version\":\"1.0\"}"
  Bus Element Out2 : Outport  PortName=ModeCommand
  Bus Element Out1 : Outport  Port=2  PortName=PilotCommand
  wires:
  Bus Element In1/1 -> ModeSelector/1(FlightCommands)
  ModeSelector/1(ModeCommand) -> Bus Element Out2/1
  Bus Element In2/1 -> CommandFormatter/1(FlightCommands)
  CommandFormatter/1(PilotCommand) -> Bus Element Out1/1

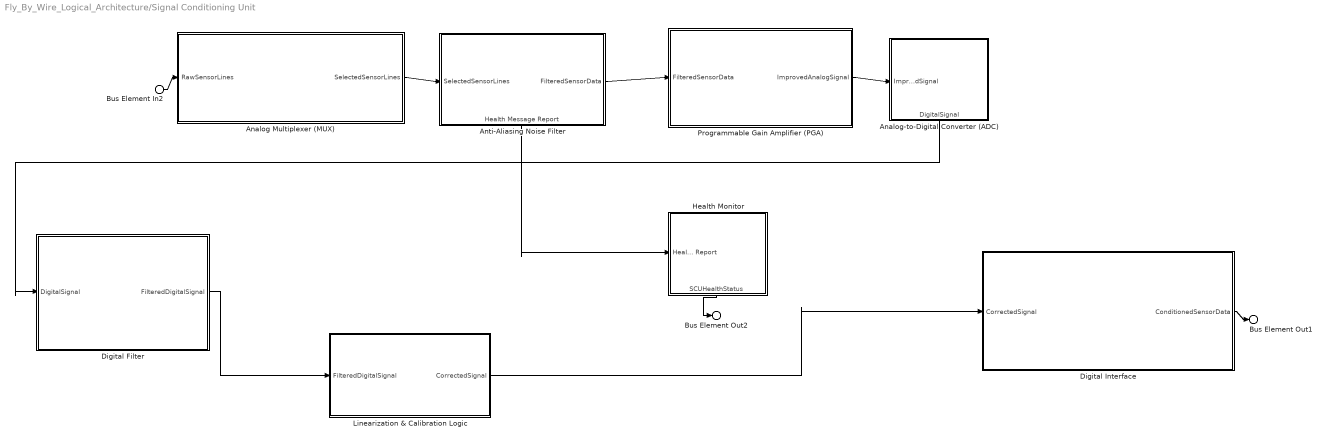
== system Fly_By_Wire_Logical_Architecture/Signal Conditioning Unit ==
  Bus Element In2 : Inport  PortName=RawSensorLines
  Analog Multiplexer (MUX) : Subsystem
      settings: PortSchema="{\"entries\":[{\"content\":{\"headerSize\":26,\"margin\":15,\"minimumSpacing\":25,\"sides\":[{\"content\":{\"connectorIds\":[\"In1\"]},\"type\":\"ConnectorPlacement.EquallySpacedRectSide\",\"uuid\":\"ba076da3-00e0-45ec-8905-3337491584c0\"},{\"content\":{\"connectorIds\":[\"Out1\"],\"side\":\"RIGHT\"},\"type\":\"ConnectorPlacement.EquallySpacedRectSide\",\"uuid\":\"72ac928f-e9a5-49d3-a941-8254f9ba21ee\"},{\"content\":{\"side\":\"TOP\"},\"type\":\"ConnectorPlacement.EquallySpacedRectSide\",\"uuid\":\"2a7ce638-5f70-4cef-9a31-c53717642639\"}]},\"type\":\"ConnectorPlacement.EquallySpacedConnector\",\"uuid\":\"ee460f65-3357-4135-aa65-636d7831ce3e\"}],\"packageUris\":[\"http://schema.mathworks.com/mf0/Connector/R2020b\"],\"version\":\"1.0\"}"
  Analog-to-Digital Converter (ADC) : Subsystem
      settings: PortSchema="{\"entries\":[{\"content\":{\"headerSize\":26,\"margin\":15,\"minimumSpacing\":25,\"sides\":[{\"content\":{\"connectorIds\":[\"In1\"]},\"type\":\"ConnectorPlacement.EquallySpacedRectSide\",\"uuid\":\"ba076da3-00e0-45ec-8905-3337491584c0\"},{\"content\":{\"side\":\"RIGHT\"},\"type\":\"ConnectorPlacement.EquallySpacedRectSide\",\"uuid\":\"72ac928f-e9a5-49d3-a941-8254f9ba21ee\"},{\"content\":{\"side\":\"TOP\"},\"type\":\"ConnectorPlacement.EquallySpacedRectSide\",\"uuid\":\"2a7ce638-5f70-4cef-9a31-c53717642639\"},{\"content\":{\"connectorIds\":[\"Out1\"],\"side\":\"BOTTOM\"},\"type\":\"ConnectorPlacement.EquallySpacedRectSide\",\"uuid\":\"0dfd022d-035b-404f-b681-8222eaabc0d9\"}]},\"type\":\"ConnectorPlacement.EquallySpacedConnector\",\"uuid\":\"ee460f65-3357-4135-aa65-636d7831ce3e\"}],\"packageUris\":[\"http://schema.mathworks.com/mf0/Connector/R2020b\"],\"version\":\"1.0\"}"
  Anti-Aliasing Noise Filter : Subsystem
      settings: PortSchema="{\"entries\":[{\"content\":{\"headerSize\":26,\"margin\":15,\"minimumSpacing\":25,\"sides\":[{\"content\":{\"connectorIds\":[\"In1\"]},\"type\":\"ConnectorPlacement.EquallySpacedRectSide\",\"uuid\":\"ba076da3-00e0-45ec-8905-3337491584c0\"},{\"content\":{\"connectorIds\":[\"Out2\"],\"side\":\"RIGHT\"},\"type\":\"ConnectorPlacement.EquallySpacedRectSide\",\"uuid\":\"72ac928f-e9a5-49d3-a941-8254f9ba21ee\"},{\"content\":{\"side\":\"TOP\"},\"type\":\"ConnectorPlacement.EquallySpacedRectSide\",\"uuid\":\"2a7ce638-5f70-4cef-9a31-c53717642639\"},{\"content\":{\"connectorIds\":[\"Out1\"],\"side\":\"BOTTOM\"},\"type\":\"ConnectorPlacement.EquallySpacedRectSide\",\"uuid\":\"30e98d84-2150-4034-bdc3-d0b6382451e0\"}]},\"type\":\"ConnectorPlacement.EquallySpacedConnector\",\"uuid\":\"ee460f65-3357-4135-aa65-636d7831ce3e\"}],\"packageUris\":[\"http://schema.mathworks.com/mf0/Connector/R2020b\"],\"version\":\"1.0\"}"
  Digital Filter : Subsystem
      settings: PortSchema="{\"entries\":[{\"content\":{\"headerSize\":26,\"margin\":15,\"minimumSpacing\":25,\"sides\":[{\"content\":{\"connectorIds\":[\"In1\"]},\"type\":\"ConnectorPlacement.EquallySpacedRectSide\",\"uuid\":\"ba076da3-00e0-45ec-8905-3337491584c0\"},{\"content\":{\"connectorIds\":[\"Out1\"],\"side\":\"RIGHT\"},\"type\":\"ConnectorPlacement.EquallySpacedRectSide\",\"uuid\":\"72ac928f-e9a5-49d3-a941-8254f9ba21ee\"},{\"content\":{\"side\":\"TOP\"},\"type\":\"ConnectorPlacement.EquallySpacedRectSide\",\"uuid\":\"2a7ce638-5f70-4cef-9a31-c53717642639\"}]},\"type\":\"ConnectorPlacement.EquallySpacedConnector\",\"uuid\":\"ee460f65-3357-4135-aa65-636d7831ce3e\"}],\"packageUris\":[\"http://schema.mathworks.com/mf0/Connector/R2020b\"],\"version\":\"1.0\"}"
  "Digital Interface " : Subsystem
      settings: PortSchema="{\"entries\":[{\"content\":{\"headerSize\":26,\"margin\":15,\"minimumSpacing\":25,\"sides\":[{\"content\":{\"connectorIds\":[\"In1\"]},\"type\":\"ConnectorPlacement.EquallySpacedRectSide\",\"uuid\":\"ba076da3-00e0-45ec-8905-3337491584c0\"},{\"content\":{\"connectorIds\":[\"Out1\"],\"side\":\"RIGHT\"},\"type\":\"ConnectorPlacement.EquallySpacedRectSide\",\"uuid\":\"72ac928f-e9a5-49d3-a941-8254f9ba21ee\"},{\"content\":{\"side\":\"TOP\"},\"type\":\"ConnectorPlacement.EquallySpacedRectSide\",\"uuid\":\"2a7ce638-5f70-4cef-9a31-c53717642639\"}]},\"type\":\"ConnectorPlacement.EquallySpacedConnector\",\"uuid\":\"ee460f65-3357-4135-aa65-636d7831ce3e\"}],\"packageUris\":[\"http://schema.mathworks.com/mf0/Connector/R2020b\"],\"version\":\"1.0\"}"
  Health Monitor : Subsystem
      settings: PortSchema="{\"entries\":[{\"content\":{\"headerSize\":26,\"margin\":15,\"minimumSpacing\":25,\"sides\":[{\"content\":{\"connectorIds\":[\"In1\"]},\"type\":\"ConnectorPlacement.EquallySpacedRectSide\",\"uuid\":\"ba076da3-00e0-45ec-8905-3337491584c0\"},{\"content\":{\"side\":\"RIGHT\"},\"type\":\"ConnectorPlacement.EquallySpacedRectSide\",\"uuid\":\"72ac928f-e9a5-49d3-a941-8254f9ba21ee\"},{\"content\":{\"side\":\"TOP\"},\"type\":\"ConnectorPlacement.EquallySpacedRectSide\",\"uuid\":\"2a7ce638-5f70-4cef-9a31-c53717642639\"},{\"content\":{\"connectorIds\":[\"Out1\"],\"side\":\"BOTTOM\"},\"type\":\"ConnectorPlacement.EquallySpacedRectSide\",\"uuid\":\"449a51f6-91d5-4038-b014-12e9eeb3d3e9\"}]},\"type\":\"ConnectorPlacement.EquallySpacedConnector\",\"uuid\":\"ee460f65-3357-4135-aa65-636d7831ce3e\"}],\"packageUris\":[\"http://schema.mathworks.com/mf0/Connector/R2020b\"],\"version\":\"1.0\"}"
  Linearization & Calibration Logic : Subsystem
      settings: PortSchema="{\"entries\":[{\"content\":{\"headerSize\":26,\"margin\":15,\"minimumSpacing\":25,\"sides\":[{\"content\":{\"connectorIds\":[\"In1\"]},\"type\":\"ConnectorPlacement.EquallySpacedRectSide\",\"uuid\":\"ba076da3-00e0-45ec-8905-3337491584c0\"},{\"content\":{\"connectorIds\":[\"Out1\"],\"side\":\"RIGHT\"},\"type\":\"ConnectorPlacement.EquallySpacedRectSide\",\"uuid\":\"72ac928f-e9a5-49d3-a941-8254f9ba21ee\"},{\"content\":{\"side\":\"TOP\"},\"type\":\"ConnectorPlacement.EquallySpacedRectSide\",\"uuid\":\"2a7ce638-5f70-4cef-9a31-c53717642639\"}]},\"type\":\"ConnectorPlacement.EquallySpacedConnector\",\"uuid\":\"ee460f65-3357-4135-aa65-636d7831ce3e\"}],\"packageUris\":[\"http://schema.mathworks.com/mf0/Connector/R2020b\"],\"version\":\"1.0\"}"
  Programmable Gain Amplifier (PGA) : Subsystem
      settings: PortSchema="{\"entries\":[{\"content\":{\"headerSize\":26,\"margin\":15,\"minimumSpacing\":25,\"sides\":[{\"content\":{\"connectorIds\":[\"In1\"]},\"type\":\"ConnectorPlacement.EquallySpacedRectSide\",\"uuid\":\"ba076da3-00e0-45ec-8905-3337491584c0\"},{\"content\":{\"connectorIds\":[\"Out1\"],\"side\":\"RIGHT\"},\"type\":\"ConnectorPlacement.EquallySpacedRectSide\",\"uuid\":\"72ac928f-e9a5-49d3-a941-8254f9ba21ee\"},{\"content\":{\"side\":\"TOP\"},\"type\":\"ConnectorPlacement.EquallySpacedRectSide\",\"uuid\":\"2a7ce638-5f70-4cef-9a31-c53717642639\"}]},\"type\":\"ConnectorPlacement.EquallySpacedConnector\",\"uuid\":\"ee460f65-3357-4135-aa65-636d7831ce3e\"}],\"packageUris\":[\"http://schema.mathworks.com/mf0/Connector/R2020b\"],\"version\":\"1.0\"}"
  Bus Element Out2 : Outport  PortName=SCUHealthStatus
  Bus Element Out1 : Outport  Port=2  PortName=ConditionedSensorData
  wires:
  Bus Element In2/1 -> Analog Multiplexer (MUX)/1(RawSensorLines)
  Analog Multiplexer (MUX)/1(SelectedSensorLines) -> Anti-Aliasing Noise Filter/1(SelectedSensorLines)
  Anti-Aliasing Noise Filter/2(FilteredSensorData) -> Programmable Gain Amplifier (PGA)/1(FilteredSensorData)
  Anti-Aliasing Noise Filter/1(Health Message Report) -> Health Monitor/1(Health Message Report)
  Programmable Gain Amplifier (PGA)/1(ImprovedAnalogSignal) -> Analog-to-Digital Converter (ADC)/1(ImprovedSignal)
  Analog-to-Digital Converter (ADC)/1(DigitalSignal) -> Digital Filter/1(DigitalSignal)
  Digital Filter/1(FilteredDigitalSignal) -> Linearization & Calibration Logic/1(FilteredDigitalSignal)
  Linearization & Calibration Logic/1(CorrectedSignal) -> "Digital Interface "/1(CorrectedSignal)
  "Digital Interface "/1(ConditionedSensorData) -> Bus Element Out1/1
  Health Monitor/1(SCUHealthStatus) -> Bus Element Out2/1

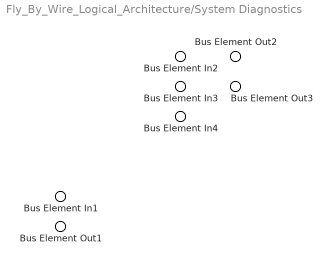
== system Fly_By_Wire_Logical_Architecture/System Diagnostics ==
  Bus Element In2 : Inport  PortName=ComplianceStatus
  Bus Element In4 : Inport  Port=2  PortName=ActuatorHealthStatus
  Bus Element In3 : Inport  Port=3  PortName=SCUHealthStatus
  Bus Element In1 : Inport  Port=4  PortName=FCPHealthReport
  Bus Element Out3 : Outport  PortName=CertificationReport
  Bus Element Out2 : Outport  Port=2  PortName=DiagnosticsReport
  Bus Element Out1 : Outport  Port=3  PortName=SelfTestCommand

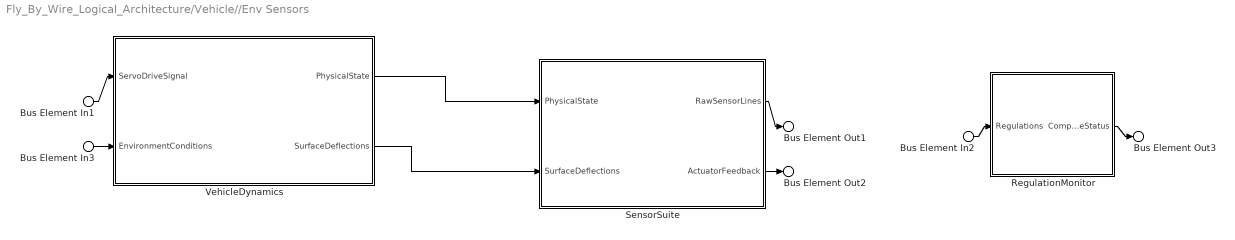
== system Fly_By_Wire_Logical_Architecture/Vehicle//Env Sensors ==
  Bus Element In2 : Inport  PortName=Regulations
  Bus Element In3 : Inport  Port=2  PortName=EnvironmentConditions
  Bus Element In1 : Inport  Port=3  PortName=ServoDriveSignal
  RegulationMonitor : Subsystem
      settings: PortSchema="{\"entries\":[{\"content\":{\"headerSize\":26,\"margin\":15,\"minimumSpacing\":25,\"sides\":[{\"content\":{\"connectorIds\":[\"In1\"]},\"type\":\"ConnectorPlacement.EquallySpacedRectSide\",\"uuid\":\"ba076da3-00e0-45ec-8905-3337491584c0\"},{\"content\":{\"connectorIds\":[\"Out1\"],\"side\":\"RIGHT\"},\"type\":\"ConnectorPlacement.EquallySpacedRectSide\",\"uuid\":\"72ac928f-e9a5-49d3-a941-8254f9ba21ee\"},{\"content\":{\"side\":\"TOP\"},\"type\":\"ConnectorPlacement.EquallySpacedRectSide\",\"uuid\":\"2a7ce638-5f70-4cef-9a31-c53717642639\"}]},\"type\":\"ConnectorPlacement.EquallySpacedConnector\",\"uuid\":\"ee460f65-3357-4135-aa65-636d7831ce3e\"}],\"packageUris\":[\"http://schema.mathworks.com/mf0/Connector/R2020b\"],\"version\":\"1.0\"}"
  SensorSuite : Subsystem
      settings: PortSchema="{\"entries\":[{\"content\":{\"headerSize\":26,\"margin\":15,\"minimumSpacing\":25,\"sides\":[{\"content\":{\"connectorIds\":[\"In1\",\"In2\"]},\"type\":\"ConnectorPlacement.EquallySpacedRectSide\",\"uuid\":\"ba076da3-00e0-45ec-8905-3337491584c0\"},{\"content\":{\"connectorIds\":[\"Out1\",\"Out2\"],\"side\":\"RIGHT\"},\"type\":\"ConnectorPlacement.EquallySpacedRectSide\",\"uuid\":\"72ac928f-e9a5-49d3-a941-8254f9ba21ee\"},{\"content\":{\"side\":\"TOP\"},\"type\":\"ConnectorPlacement.EquallySpacedRectSide\",\"uuid\":\"2a7ce638-5f70-4cef-9a31-c53717642639\"}]},\"type\":\"ConnectorPlacement.EquallySpacedConnector\",\"uuid\":\"ee460f65-3357-4135-aa65-636d7831ce3e\"}],\"packageUris\":[\"http://schema.mathworks.com/mf0/Connector/R2020b\"],\"version\":\"1.0\"}"
  VehicleDynamics : Subsystem
      settings: PortSchema="{\"entries\":[{\"content\":{\"headerSize\":26,\"margin\":15,\"minimumSpacing\":25,\"sides\":[{\"content\":{\"connectorIds\":[\"In1\",\"In2\"]},\"type\":\"ConnectorPlacement.EquallySpacedRectSide\",\"uuid\":\"ba076da3-00e0-45ec-8905-3337491584c0\"},{\"content\":{\"connectorIds\":[\"Out1\",\"Out2\"],\"side\":\"RIGHT\"},\"type\":\"ConnectorPlacement.EquallySpacedRectSide\",\"uuid\":\"72ac928f-e9a5-49d3-a941-8254f9ba21ee\"},{\"content\":{\"side\":\"TOP\"},\"type\":\"ConnectorPlacement.EquallySpacedRectSide\",\"uuid\":\"2a7ce638-5f70-4cef-9a31-c53717642639\"}]},\"type\":\"ConnectorPlacement.EquallySpacedConnector\",\"uuid\":\"ee460f65-3357-4135-aa65-636d7831ce3e\"}],\"packageUris\":[\"http://schema.mathworks.com/mf0/Connector/R2020b\"],\"version\":\"1.0\"}"
  Bus Element Out3 : Outport  PortName=ComplianceStatus
  Bus Element Out1 : Outport  Port=2  PortName=RawSensorLines
  Bus Element Out2 : Outport  Port=3  PortName=ActuatorFeedback
  wires:
  Bus Element In1/1 -> VehicleDynamics/1(ServoDriveSignal)
  Bus Element In3/1 -> VehicleDynamics/2(EnvironmentConditions)
  VehicleDynamics/1(PhysicalState) -> SensorSuite/1(PhysicalState)
  VehicleDynamics/2(SurfaceDeflections) -> SensorSuite/2(SurfaceDeflections)
  SensorSuite/1(RawSensorLines) -> Bus Element Out1/1
  SensorSuite/2(ActuatorFeedback) -> Bus Element Out2/1
  Bus Element In2/1 -> RegulationMonitor/1(Regulations)
  RegulationMonitor/1(ComplianceStatus) -> Bus Element Out3/1

== system Fly_By_Wire_Logical_Architecture/Actuator Interface/Actuation Bus ==
  Bus Element In1 : Inport  PortName=SpoilerDrive
  Bus Element In2 : Inport  Port=2  PortName=ElevatorDruver
  Bus Element In3 : Inport  Port=3  PortName=RudderDrive
  Bus Element In4 : Inport  Port=4  PortName=AileronDrive
  Bus Element Out1 : Outport  PortName=ServoDriveSignal

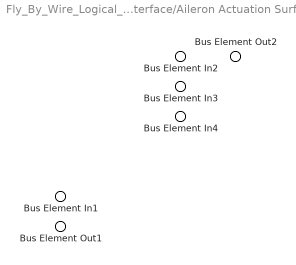
== system Fly_By_Wire_Logical_Architecture/Actuator Interface/Aileron Actuation Surface ==
  Bus Element In2 : Inport  PortName=AileronActuationCommand
  Bus Element In3 : Inport  Port=2  PortName=ConfigCommand
  Bus Element In4 : Inport  Port=3  PortName=SelfTestCommand
  Bus Element In1 : Inport  Port=4  PortName=ActuatorFeedback
  Bus Element Out2 : Outport  PortName=AileronChannelHealthMessage
  Bus Element Out1 : Outport  Port=2  PortName=AileronDrive

== system Fly_By_Wire_Logical_Architecture/Actuator Interface/Command Demultiplexer ==
  Bus Element In1 : Inport  PortName=ActuatorDriveSignal
  Bus Element Out2 : Outport  PortName=AileronActuationCommand
  Bus Element Out3 : Outport  Port=2  PortName=RudderActuationCommand
  Bus Element Out1 : Outport  Port=3  PortName=ElevatorActuationCommand
  Bus Element Out4 : Outport  Port=4  PortName=SpoilerActuationCommand

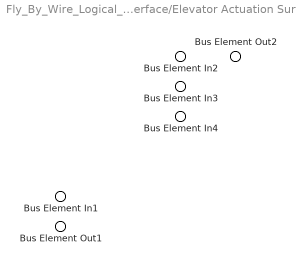
== system Fly_By_Wire_Logical_Architecture/Actuator Interface/Elevator Actuation Surface ==
  Bus Element In2 : Inport  PortName=ElevatorActuationCommand
  Bus Element In3 : Inport  Port=2  PortName=ConfigCommand
  Bus Element In4 : Inport  Port=3  PortName=SelfTestCommand
  Bus Element In1 : Inport  Port=4  PortName=ActuatorFeedback
  Bus Element Out2 : Outport  PortName=ElevatorChannelHealthMessage
  Bus Element Out1 : Outport  Port=2  PortName=ElevatorDriver

== system Fly_By_Wire_Logical_Architecture/Actuator Interface/Health Aggregator ==
  Bus Element In4 : Inport  PortName=AileronChannelHealthMessage
  Bus Element In3 : Inport  Port=2  PortName=RudderChannelHealthMessage
  Bus Element In2 : Inport  Port=3  PortName=ElevatorChannelHealthMessage
  Bus Element In1 : Inport  Port=4  PortName=SpoilerChannelHealthMessage
  Bus Element Out1 : Outport  PortName=ActuatorHealthStatus

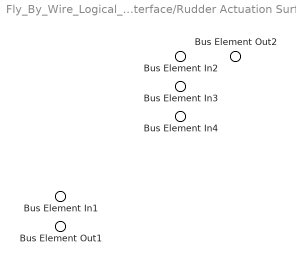
== system Fly_By_Wire_Logical_Architecture/Actuator Interface/Rudder Actuation Surface ==
  Bus Element In2 : Inport  PortName=RudderActuationCommand
  Bus Element In3 : Inport  Port=2  PortName=ConfigCommand
  Bus Element In4 : Inport  Port=3  PortName=SelfTestCommand
  Bus Element In1 : Inport  Port=4  PortName=ActuatorFeedback
  Bus Element Out2 : Outport  PortName=RudderChannelHealthMessage
  Bus Element Out1 : Outport  Port=2  PortName=RudderDrive

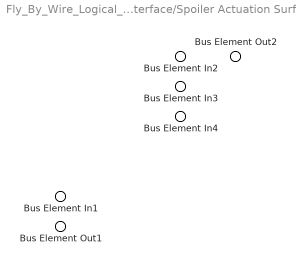
== system Fly_By_Wire_Logical_Architecture/Actuator Interface/Spoiler Actuation Surface ==
  Bus Element In2 : Inport  PortName=SpoilerActuationCommand
  Bus Element In3 : Inport  Port=2  PortName=ConfigCommand
  Bus Element In4 : Inport  Port=3  PortName=SelfTestCommand
  Bus Element In1 : Inport  Port=4  PortName=ActuatorFeedback
  Bus Element Out2 : Outport  PortName=ChannelsHealthMessage
  Bus Element Out1 : Outport  Port=2  PortName=SpoilerDrive

== system Fly_By_Wire_Logical_Architecture/Autopilot Manager/Command Arbitrator ==
  Bus Element In2 : Inport  PortName=SafeAutoCommand
  Bus Element In1 : Inport  Port=2  PortName=autoEnabled
  Bus Element Out1 : Outport  PortName=AutoCommand

== system Fly_By_Wire_Logical_Architecture/Autopilot Manager/Envelope Protector ==
  Bus Element In1 : Inport  PortName=InitialAutocommand
  Bus Element Out1 : Outport  PortName=SafeAutoCommand
